simulink model "pidcontrol"  (R2013a)
settings: Solver=ode4  StartTime=0.0  StopTime=10  FixedStep=1e-4  RelTol=1e-3
libraries: simulink x1
settings Model: Creator=ugurm  LastModifiedBy=ugurm

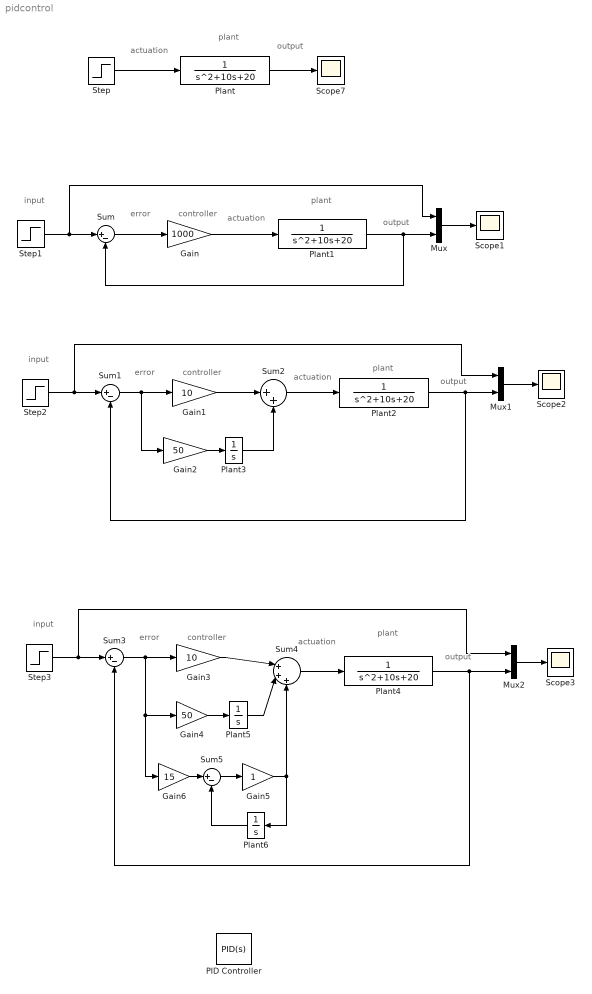
== system pidcontrol ==
  note: error
  note: actuation
  note: output
  note: controller
  note: plant
  note: plant
  note: actuation
  note: output
  note: input
  note: error
  note: controller
  note: plant
  note: actuation
  note: output
  note: input
  note: error
  note: controller
  note: plant
  note: actuation
  note: output
  note: input
  Gain : Gain  Gain=1000
  Gain1 : Gain  Gain=10
  Gain2 : Gain  Gain=50
  Gain3 : Gain  Gain=10
  Gain4 : Gain  Gain=50
  Gain5 : Gain
  Gain6 : Gain  Gain=15
  Mux : Mux  Inputs=2
  Mux1 : Mux  Inputs=2
  Mux2 : Mux  Inputs=2
  PID Controller : simulink/Continuous/PID Controller  Controller=PID  TimeDomain=Continuous-time  SampleTime=1  IntegratorMethod=Forward Euler  FilterMethod=Forward Euler  Form=Parallel  P=1  I=1  D=0  N=100  InitialConditionSource=internal  InitialConditionForIntegrator=0  InitialConditionForFilter=0  ExternalReset=none  LimitOutput=off  UpperSaturationLimit=inf  LowerSaturationLimit=-inf  LinearizeAsGain=on  AntiWindupMode=none  Kb=1  TrackingMode=off  Kt=1  PParamMin=[]  PParamMax=[]  IParamMin=[]  IParamMax=[]  DParamMin=[]  DParamMax=[]  NParamMin=[]  NParamMax=[]  KbParamMin=[]  KbParamMax=[]  KtParamMin=[]  KtParamMax=[]  POutMin=[]  POutMax=[]  IOutMin=[]  IOutMax=[]  DOutMin=[]  DOutMax=[]  NOutMin=[]  NOutMax=[]  KbOutMin=[]  KbOutMax=[]  KtOutMin=[]  KtOutMax=[]  IntegratorOutMin=[]  IntegratorOutMax=[]  FilterOutMin=[]  FilterOutMax=[]  SumOutMin=[]  SumOutMax=[]  SumI1OutMin=[]  SumI1OutMax=[]  SumI2OutMin=[]  SumI2OutMax=[]  SumI3OutMin=[]  SumI3OutMax=[]  SumDOutMin=[]  SumDOutMax=[]  SaturationOutMin=[]  SaturationOutMax=[]  IntegratorContinuousStateAttributes=''  IntegratorStateMustResolveToSignalObject=off  IntegratorRTWStateStorageClass=Auto  FilterContinuousStateAttributes=''  FilterStateMustResolveToSignalObject=off  FilterRTWStateStorageClass=Auto
  Plant{,1..2,4} (4 alike) : TransferFcn  Denominator=[1 10 20]
  Plant3 : TransferFcn  Denominator=[1 0]
  Plant5 : TransferFcn  Denominator=[1 0]
  Plant6 : TransferFcn  Denominator=[1 0]
  Scope{1..3,7} (4 alike) : Scope
      Scope1 settings: YMin=0  YMax=430
      Scope2 settings: YMin=0  YMax=1.1
      Scope3 settings: YMin=0  YMax=1.1  SaveName=ScopeData2
      Scope7 settings: YMin=0  YMax=430  SaveName=ScopeData6
  Step{,1..3} (4 alike) : Step  Time=0.2  SampleTime=0
  Sum{,1,3,5} (4 alike) : Sum  Inputs=|+-
  Sum2 : Sum  Inputs=|++
  Sum4 : Sum  Inputs=|+++
  wires:
  Step/1 -> Plant/1
  Plant/1 -> Scope7/1
  Gain/1 -> Plant1/1
  Sum/1 -> Gain/1
  Plant1/1 -> Mux/2, Sum/2
  Step1/1 -> Mux/1, Sum/1
  Mux/1 -> Scope1/1
  Sum1/1 -> Gain2/1, Gain1/1
  Plant2/1 -> Mux1/2, Sum1/2
  Step2/1 -> Mux1/1, Sum1/1
  Mux1/1 -> Scope2/1
  Sum2/1 -> Plant2/1
  Gain2/1 -> Plant3/1
  Gain1/1 -> Sum2/1
  Plant3/1 -> Sum2/2
  Plant4/1 -> Mux2/2, Sum3/2
  Step3/1 -> Mux2/1, Sum3/1
  Mux2/1 -> Scope3/1
  Sum4/1 -> Plant4/1
  Gain4/1 -> Plant5/1
  Gain3/1 -> Sum4/1
  Plant5/1 -> Sum4/2
  Gain5/1 -> Sum4/3, Plant6/1
  Sum5/1 -> Gain5/1
  Sum3/1 -> Gain6/1, Gain4/1, Gain3/1
  Plant6/1 -> Sum5/2
  Gain6/1 -> Sum5/1
